simulink model "sim_ROV_v0_R2018b"  (R2023a)
settings: Solver=ode4  StartTime=0.0  StopTime=sim_time  FixedStep=Ts  RelTol=1e-3
values from neighbouring files (symbols this model uses):
  B = rho*V*g*1.4    (= 168.9282)    [launcher_ROV_sim.m]    (also in lqr_design.m = [0.05581,         0,         0,         0,         0,       )
  D_linear = diag([D_u, D_v, D_w, D_p, D_q, D_r])    [launcher_ROV_sim.m]
  D_quadratic = diag([D_uu, D_vv, D_ww, D_pp, D_qq, D_rr])    [launcher_ROV_sim.m]
  force = lookup.Force_14V_Kgf    [launcher_ROV_sim.m]
  I = [I_xx   -I_xy   -I_xz ... (first row only)    [launcher_ROV_sim.m]
  Kq = [-14.0522937866 -0.000724361189881 7.36173354264e-14 -0.00802187271501 -1.59153029576 -0.00240388685004 -0.00102573418256 -14.0209983601 3.7395785387e-14 1.84702452338 0.00611607698573 0.00818162190067 ... (36 elements, 6x6)]    [lqr.mat]    (also in lqr_design.m = K(:,13:end))
  Kx = [30.0077125539 0.00159520383282 -9.18372190817e-14 0.0101724452135 3.59932945814 0.00293162043647 0.00170650423442 25.0803818094 -2.91671924306e-14 -3.06896094423 -0.00658141948351 -0.00836683203268 ... (72 elements, 6x12)]    [lqr.mat]    (also in lqr_design.m = K(:,1:12))
  m = 16.6    [launcher_ROV_sim.m]
  M_addedMass = [1.3169    0         0         0         0         0 ... (first row only)    [launcher_ROV_sim.m]
  M_rigidBody = [m        0        0        0          m*z_g     -m*y_g ... (first row only)    [launcher_ROV_sim.m]
  pwm = lookup.PWM    [launcher_ROV_sim.m]
  r_b = [x_b y_b z_b]'    [launcher_ROV_sim.m]
  r_g = [x_g y_g z_g]'    [launcher_ROV_sim.m]
  sim_time = 100    [launcher_ROV_sim.m]    (also in lqr_design.m)
  TCM = [ -0.7071   -0.7071    0.7071    0.7071    0         0         0         0 ... (first row only)    [launcher_ROV_sim.m]
  Ts = 0.01    [launcher_ROV_sim.m]    (also in lqr_design.m)
  W = m*g    (= 162.846)    [launcher_ROV_sim.m]
libraries: slpidlib x6, dspfdesign x6, simulink x2, aerolibnav x1, sharedtransform x1, aerolibanim x1
(part 1 of 2)
settings Model: SimulationMode=accelerator  Creator=d066103  LastModifiedBy=retr0
settings SolverCC: AlgebraicLoopSolver=TrustRegion
settings DataIOCC: ReturnWorkspaceOutputs=off
settings DebuggingCC: UnconnectedInputMsg=warning  UnconnectedOutputMsg=warning  UnconnectedLineMsg=warning  ArithmeticOperatorsInVariantConditions=warning
settings HardwareCC: ProdBitPerPointer=32  ProdBitPerSizeT=32  ProdBitPerPtrDiffT=32  ProdLargestAtomicInteger=Long  ProdLargestAtomicFloat=Double  ProdWordSize=32  ProdHWDeviceType=ARM Compatible->ARM Cortex-M
settings ModelReferenceCC: EnableRefExpFcnMdlSchedulingChecks=on
settings SFSimCC: CustomCodeUndefinedFunction=UseInterfaceOnly
settings RTWCC: PackageGeneratedCodeAndArtifacts=on  TargetLang=C++
settings GRTTargetCC: TargetLangStandard=C++11 (ISO)

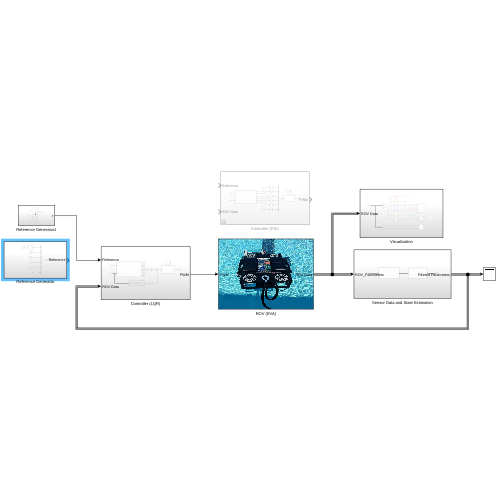
[thumbnail: Simulink's stored preview of the top-level diagram]
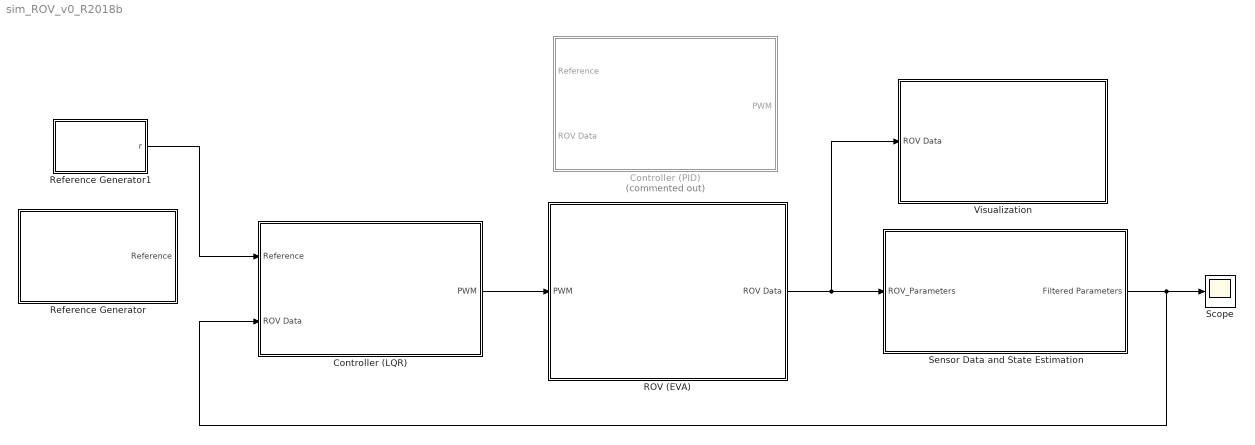
== system sim_ROV_v0_R2018b ==
  Controller (LQR) : Subsystem
  Controller (PID) : Subsystem  Commented=on
  ROV (EVA) : Subsystem
      mask Display: image('eva.jpg');
  Reference Generator : Subsystem
  Reference Generator1 : Subsystem
  Scope : Scope
  Sensor Data and State Estimation : Subsystem
  Visualization : Subsystem
  wires:
  ROV (EVA)/1(ROV Data) -> Visualization/1(ROV Data), Sensor Data and State Estimation/1(ROV_Parameters)
  Reference Generator1/1(r) -> Controller (LQR)/1(Reference)
  Controller (LQR)/1(PWM) -> ROV (EVA)/1(PWM)
  Sensor Data and State Estimation/1(Filtered Parameters) -> Scope/1, Controller (LQR)/2(ROV Data)

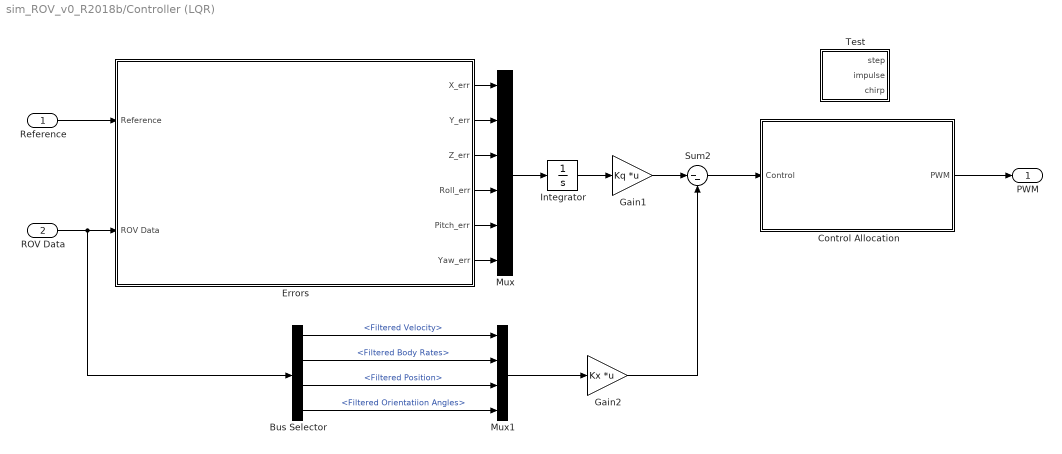
== system sim_ROV_v0_R2018b/Controller (LQR) ==
  Reference : Inport
  ROV Data : Inport  Port=2
  Bus Selector : BusSelector  OutputSignals=Filtered Velocity,Filtered Body Rates,Filtered Position,Filtered Orientatiion Angles
  Control Allocation : Subsystem
  Errors : Subsystem
  Gain1 : Gain  Gain=Kq  Multiplication=Matrix(K*u)
  Gain2 : Gain  Gain=Kx  Multiplication=Matrix(K*u)
  Integrator : Integrator
  Mux : Mux  Inputs=6
  Mux1 : Mux
  Sum2 : Sum  Inputs=|--
  Test : Subsystem
  PWM : Outport  VectorParamsAs1DForOutWhenUnconnected=off
  wires:
  Control Allocation/1(PWM) -> PWM/1
  Reference/1 -> Errors/1(Reference)
  ROV Data/1 -> Bus Selector/1, Errors/2(ROV Data)
  Errors/6(Yaw_err) -> Mux/6
  Errors/5(Pitch_err) -> Mux/5
  Errors/4(Roll_err) -> Mux/4
  Errors/3(Z_err) -> Mux/3
  Errors/2(Y_err) -> Mux/2
  Errors/1(X_err) -> Mux/1
  Mux/1 -> Integrator/1
  Gain1/1 -> Sum2/1
  Sum2/1 -> Control Allocation/1(Control)
  Gain2/1 -> Sum2/2
  Mux1/1 -> Gain2/1
  Bus Selector/2 -> Mux1/2  "<Filtered Body Rates>"
  Integrator/1 -> Gain1/1
  Bus Selector/3 -> Mux1/3  "<Filtered Position>"
  Bus Selector/4 -> Mux1/4  "<Filtered Orientatiion Angles>"
  Bus Selector/1 -> Mux1/1  "<Filtered Velocity>"

== system sim_ROV_v0_R2018b/Controller (PID) ==
  Reference : Inport
  ROV Data : Inport  Port=2
  Control Allocation : Subsystem
  Controller Pitch : slpidlib/PID Controller  Controller=PID  Form=Ideal  TimeDomain=Continuous-time  UseExternalTs=off  SampleTime=-1  IntegratorMethod=Forward Euler  FilterMethod=Forward Euler  ControllerParametersSource=internal  P=137.468345289691  I=0.00452061904362843  UseKiTs=off  D=0.10598803802833  N=59.0701245414644  UseFilter=on  TunerSelectOption=Transfer Function Based (PID Tuner App)  InitialConditionSource=internal  InitialConditionForIntegrator=0  InitialConditionForFilter=0  DifferentiatorICPrevScaledInput=0  ExternalReset=none  TrackingMode=off  Kt=1  LimitOutput=off  SatLimitsSource=internal  UpperSaturationLimit=inf  LowerSaturationLimit=-inf  LinearizeAsGain=on  AntiWindupMode=none  Kb=1  LimitIntegrator=off  UpperIntegratorSaturationLimit=inf  LowerIntegratorSaturationLimit=-inf  POutMin=[]  POutMax=[]  IOutMin=[]  IOutMax=[]  DOutMin=[]  DOutMax=[]  NOutMin=[]  NOutMax=[]  SumOutMin=[]  SumOutMax=[]  SaturationOutMin=[]  SaturationOutMax=[]  PParamMin=[]  PParamMax=[]  IParamMin=[]  IParamMax=[]  DParamMin=[]  DParamMax=[]  NParamMin=[]  NParamMax=[]  KbParamMin=[]  KbParamMax=[]  KtParamMin=[]  KtParamMax=[]  KbOutMin=[]  KbOutMax=[]  KtOutMin=[]  KtOutMax=[]  IntegratorOutMin=[]  IntegratorOutMax=[]  FilterOutMin=[]  FilterOutMax=[]  SumI1OutMin=[]  SumI1OutMax=[]  SumI2OutMin=[]  SumI2OutMax=[]  SumI3OutMin=[]  SumI3OutMax=[]  SumI4OutMin=[]  SumI4OutMax=[]  SumDOutMin=[]  SumDOutMax=[]  DifferentiatorOutMin=[]  DifferentiatorOutMax=[]  FilterDiffOutCoefMin=[]  FilterDiffOutCoefMax=[]  ReciprocalOutMin=[]  ReciprocalOutMax=[]  SumDenOutMin=[]  SumDenOutMax=[]  SumNumOutMin=[]  SumNumOutMax=[]  DivideOutMin=[]  DivideOutMax=[]  UdiffTsProdOutMin=[]  UdiffTsProdOutMax=[]  NTsProdOutMin=[]  NTsProdOutMax=[]  UintegralTsProdOutMin=[]  UintegralTsProdOutMax=[]  UngainTsProdOutMin=[]  UngainTsProdOutMax=[]  ClampingZeroOutDataTypeStr=Inherit: Inherit via back propagation  ClampingZeroOutMin=[]  ClampingZeroOutMax=[]  FilterDenConstantOutDataTypeStr=Inherit: Inherit via back propagation  FilterDenConstantOutMin=[]  FilterDenConstantOutMax=[]  PCopyOutDataTypeStr=Inherit: Inherit via back propagation  PCopyOutMin=[]  PCopyOutMax=[]  NCopyOutDataTypeStr=Inherit: Inherit via back propagation  NCopyOutMin=[]  NCopyOutMax=[]  IntegratorContinuousStateAttributes=''  IntegratorStateMustResolveToSignalObject=off  IntegratorRTWStateStorageClass=Auto  FilterContinuousStateAttributes=''  FilterStateMustResolveToSignalObject=off  FilterRTWStateStorageClass=Auto  ParallelPVariant=Passthrough  IdealPVariant=InternalParameters  IVariant=InternalParameters  DVariant=InternalParameters  IntegratorVariant=Continuous  SatVariant=Disabled  AWVariant=Passthrough  PCopyVariant=Disabled  TRVariant=Disabled  FdbkBlocksVariant=Forward  IdealPFdbkVariant=Disabled  SatFdbkVariant=Disabled  DerivativeFilterVariant=ContFilter  NVariant=InternalParameters  NCopyVariant=Disabled  FilterICVariant=InternalICsFilter  IntegratorICVariant=InternalICs  ExternalResetVariant=Disabled  TRSumVariant=Passthrough  SumFdbkVariant=Disabled  SumVariant=Sum_PID  TsampFilterVariant=InternalTs  TsampNgainVariant=Passthrough  TsampIntegralVariant=Disabled_SignalSpec  ExternalSaturationOutDataTypeStr=Inherit: Same as second input
  Controller Roll : slpidlib/PID Controller  Controller=PD  Form=Ideal  TimeDomain=Continuous-time  UseExternalTs=off  SampleTime=-1  IntegratorMethod=Forward Euler  FilterMethod=Forward Euler  ControllerParametersSource=internal  P=338.734488453615  I=0.00899012295658062  UseKiTs=off  D=0.0949817527302428  N=190.888436374434  UseFilter=on  TunerSelectOption=Transfer Function Based (PID Tuner App)  InitialConditionSource=internal  InitialConditionForIntegrator=0  InitialConditionForFilter=0  DifferentiatorICPrevScaledInput=0  ExternalReset=none  TrackingMode=off  Kt=1  LimitOutput=off  SatLimitsSource=internal  UpperSaturationLimit=inf  LowerSaturationLimit=-inf  LinearizeAsGain=on  AntiWindupMode=none  Kb=1  LimitIntegrator=off  UpperIntegratorSaturationLimit=inf  LowerIntegratorSaturationLimit=-inf  POutMin=[]  POutMax=[]  IOutMin=[]  IOutMax=[]  DOutMin=[]  DOutMax=[]  NOutMin=[]  NOutMax=[]  SumOutMin=[]  SumOutMax=[]  SaturationOutMin=[]  SaturationOutMax=[]  PParamMin=[]  PParamMax=[]  IParamMin=[]  IParamMax=[]  DParamMin=[]  DParamMax=[]  NParamMin=[]  NParamMax=[]  KbParamMin=[]  KbParamMax=[]  KtParamMin=[]  KtParamMax=[]  KbOutMin=[]  KbOutMax=[]  KtOutMin=[]  KtOutMax=[]  IntegratorOutMin=[]  IntegratorOutMax=[]  FilterOutMin=[]  FilterOutMax=[]  SumI1OutMin=[]  SumI1OutMax=[]  SumI2OutMin=[]  SumI2OutMax=[]  SumI3OutMin=[]  SumI3OutMax=[]  SumI4OutMin=[]  SumI4OutMax=[]  SumDOutMin=[]  SumDOutMax=[]  DifferentiatorOutMin=[]  DifferentiatorOutMax=[]  FilterDiffOutCoefMin=[]  FilterDiffOutCoefMax=[]  ReciprocalOutMin=[]  ReciprocalOutMax=[]  SumDenOutMin=[]  SumDenOutMax=[]  SumNumOutMin=[]  SumNumOutMax=[]  DivideOutMin=[]  DivideOutMax=[]  UdiffTsProdOutMin=[]  UdiffTsProdOutMax=[]  NTsProdOutMin=[]  NTsProdOutMax=[]  UintegralTsProdOutMin=[]  UintegralTsProdOutMax=[]  UngainTsProdOutMin=[]  UngainTsProdOutMax=[]  ClampingZeroOutDataTypeStr=Inherit: Inherit via back propagation  ClampingZeroOutMin=[]  ClampingZeroOutMax=[]  FilterDenConstantOutDataTypeStr=Inherit: Inherit via back propagation  FilterDenConstantOutMin=[]  FilterDenConstantOutMax=[]  PCopyOutDataTypeStr=Inherit: Inherit via back propagation  PCopyOutMin=[]  PCopyOutMax=[]  NCopyOutDataTypeStr=Inherit: Inherit via back propagation  NCopyOutMin=[]  NCopyOutMax=[]  IntegratorContinuousStateAttributes=''  IntegratorStateMustResolveToSignalObject=off  IntegratorRTWStateStorageClass=Auto  FilterContinuousStateAttributes=''  FilterStateMustResolveToSignalObject=off  FilterRTWStateStorageClass=Auto  ParallelPVariant=Passthrough  IdealPVariant=InternalParameters  IVariant=Disabled  DVariant=InternalParameters  IntegratorVariant=Disabled  SatVariant=Disabled  AWVariant=Disabled  PCopyVariant=Disabled  TRVariant=Disabled  FdbkBlocksVariant=Forward  IdealPFdbkVariant=Disabled  SatFdbkVariant=Disabled  DerivativeFilterVariant=ContFilter  NVariant=InternalParameters  NCopyVariant=Disabled  FilterICVariant=InternalICsFilter  IntegratorICVariant=Disabled  ExternalResetVariant=Disabled  TRSumVariant=Passthrough  SumFdbkVariant=Disabled  SumVariant=Sum_PD  TsampFilterVariant=InternalTs  TsampNgainVariant=Passthrough  TsampIntegralVariant=Disabled_SignalSpec  ExternalSaturationOutDataTypeStr=Inherit: Same as second input
  Controller X : slpidlib/PID Controller  Controller=PD  Form=Ideal  TimeDomain=Continuous-time  UseExternalTs=off  SampleTime=-1  IntegratorMethod=Forward Euler  FilterMethod=Forward Euler  ControllerParametersSource=internal  P=26.505422427304  I=0.00899012295658062  UseKiTs=off  D=0.620337341254882  N=0.955497663107341  UseFilter=on  TunerSelectOption=Transfer Function Based (PID Tuner App)  InitialConditionSource=internal  InitialConditionForIntegrator=0  InitialConditionForFilter=0  DifferentiatorICPrevScaledInput=0  ExternalReset=none  TrackingMode=off  Kt=1  LimitOutput=off  SatLimitsSource=internal  UpperSaturationLimit=inf  LowerSaturationLimit=-inf  LinearizeAsGain=on  AntiWindupMode=none  Kb=1  LimitIntegrator=off  UpperIntegratorSaturationLimit=inf  LowerIntegratorSaturationLimit=-inf  POutMin=[]  POutMax=[]  IOutMin=[]  IOutMax=[]  DOutMin=[]  DOutMax=[]  NOutMin=[]  NOutMax=[]  SumOutMin=[]  SumOutMax=[]  SaturationOutMin=[]  SaturationOutMax=[]  PParamMin=[]  PParamMax=[]  IParamMin=[]  IParamMax=[]  DParamMin=[]  DParamMax=[]  NParamMin=[]  NParamMax=[]  KbParamMin=[]  KbParamMax=[]  KtParamMin=[]  KtParamMax=[]  KbOutMin=[]  KbOutMax=[]  KtOutMin=[]  KtOutMax=[]  IntegratorOutMin=[]  IntegratorOutMax=[]  FilterOutMin=[]  FilterOutMax=[]  SumI1OutMin=[]  SumI1OutMax=[]  SumI2OutMin=[]  SumI2OutMax=[]  SumI3OutMin=[]  SumI3OutMax=[]  SumI4OutMin=[]  SumI4OutMax=[]  SumDOutMin=[]  SumDOutMax=[]  DifferentiatorOutMin=[]  DifferentiatorOutMax=[]  FilterDiffOutCoefMin=[]  FilterDiffOutCoefMax=[]  ReciprocalOutMin=[]  ReciprocalOutMax=[]  SumDenOutMin=[]  SumDenOutMax=[]  SumNumOutMin=[]  SumNumOutMax=[]  DivideOutMin=[]  DivideOutMax=[]  UdiffTsProdOutMin=[]  UdiffTsProdOutMax=[]  NTsProdOutMin=[]  NTsProdOutMax=[]  UintegralTsProdOutMin=[]  UintegralTsProdOutMax=[]  UngainTsProdOutMin=[]  UngainTsProdOutMax=[]  ClampingZeroOutDataTypeStr=Inherit: Inherit via back propagation  ClampingZeroOutMin=[]  ClampingZeroOutMax=[]  FilterDenConstantOutDataTypeStr=Inherit: Inherit via back propagation  FilterDenConstantOutMin=[]  FilterDenConstantOutMax=[]  PCopyOutDataTypeStr=Inherit: Inherit via back propagation  PCopyOutMin=[]  PCopyOutMax=[]  NCopyOutDataTypeStr=Inherit: Inherit via back propagation  NCopyOutMin=[]  NCopyOutMax=[]  IntegratorContinuousStateAttributes=''  IntegratorStateMustResolveToSignalObject=off  IntegratorRTWStateStorageClass=Auto  FilterContinuousStateAttributes=''  FilterStateMustResolveToSignalObject=off  FilterRTWStateStorageClass=Auto  ParallelPVariant=Passthrough  IdealPVariant=InternalParameters  IVariant=Disabled  DVariant=InternalParameters  IntegratorVariant=Disabled  SatVariant=Disabled  AWVariant=Disabled  PCopyVariant=Disabled  TRVariant=Disabled  FdbkBlocksVariant=Forward  IdealPFdbkVariant=Disabled  SatFdbkVariant=Disabled  DerivativeFilterVariant=ContFilter  NVariant=InternalParameters  NCopyVariant=Disabled  FilterICVariant=InternalICsFilter  IntegratorICVariant=Disabled  ExternalResetVariant=Disabled  TRSumVariant=Passthrough  SumFdbkVariant=Disabled  SumVariant=Sum_PD  TsampFilterVariant=InternalTs  TsampNgainVariant=Passthrough  TsampIntegralVariant=Disabled_SignalSpec  ExternalSaturationOutDataTypeStr=Inherit: Same as second input
  Controller Y : slpidlib/PID Controller  Controller=PD  Form=Ideal  TimeDomain=Continuous-time  UseExternalTs=off  SampleTime=-1  IntegratorMethod=Forward Euler  FilterMethod=Forward Euler  ControllerParametersSource=internal  P=54.0411515772124  I=0.00335999548481141  UseKiTs=off  D=3.50685578049318  N=0.462269774575205  UseFilter=on  TunerSelectOption=Transfer Function Based (PID Tuner App)  InitialConditionSource=internal  InitialConditionForIntegrator=0  InitialConditionForFilter=0  DifferentiatorICPrevScaledInput=0  ExternalReset=none  TrackingMode=off  Kt=1  LimitOutput=off  SatLimitsSource=internal  UpperSaturationLimit=inf  LowerSaturationLimit=-inf  LinearizeAsGain=on  AntiWindupMode=none  Kb=1  LimitIntegrator=off  UpperIntegratorSaturationLimit=inf  LowerIntegratorSaturationLimit=-inf  POutMin=[]  POutMax=[]  IOutMin=[]  IOutMax=[]  DOutMin=[]  DOutMax=[]  NOutMin=[]  NOutMax=[]  SumOutMin=[]  SumOutMax=[]  SaturationOutMin=[]  SaturationOutMax=[]  PParamMin=[]  PParamMax=[]  IParamMin=[]  IParamMax=[]  DParamMin=[]  DParamMax=[]  NParamMin=[]  NParamMax=[]  KbParamMin=[]  KbParamMax=[]  KtParamMin=[]  KtParamMax=[]  KbOutMin=[]  KbOutMax=[]  KtOutMin=[]  KtOutMax=[]  IntegratorOutMin=[]  IntegratorOutMax=[]  FilterOutMin=[]  FilterOutMax=[]  SumI1OutMin=[]  SumI1OutMax=[]  SumI2OutMin=[]  SumI2OutMax=[]  SumI3OutMin=[]  SumI3OutMax=[]  SumI4OutMin=[]  SumI4OutMax=[]  SumDOutMin=[]  SumDOutMax=[]  DifferentiatorOutMin=[]  DifferentiatorOutMax=[]  FilterDiffOutCoefMin=[]  FilterDiffOutCoefMax=[]  ReciprocalOutMin=[]  ReciprocalOutMax=[]  SumDenOutMin=[]  SumDenOutMax=[]  SumNumOutMin=[]  SumNumOutMax=[]  DivideOutMin=[]  DivideOutMax=[]  UdiffTsProdOutMin=[]  UdiffTsProdOutMax=[]  NTsProdOutMin=[]  NTsProdOutMax=[]  UintegralTsProdOutMin=[]  UintegralTsProdOutMax=[]  UngainTsProdOutMin=[]  UngainTsProdOutMax=[]  ClampingZeroOutDataTypeStr=Inherit: Inherit via back propagation  ClampingZeroOutMin=[]  ClampingZeroOutMax=[]  FilterDenConstantOutDataTypeStr=Inherit: Inherit via back propagation  FilterDenConstantOutMin=[]  FilterDenConstantOutMax=[]  PCopyOutDataTypeStr=Inherit: Inherit via back propagation  PCopyOutMin=[]  PCopyOutMax=[]  NCopyOutDataTypeStr=Inherit: Inherit via back propagation  NCopyOutMin=[]  NCopyOutMax=[]  IntegratorContinuousStateAttributes=''  IntegratorStateMustResolveToSignalObject=off  IntegratorRTWStateStorageClass=Auto  FilterContinuousStateAttributes=''  FilterStateMustResolveToSignalObject=off  FilterRTWStateStorageClass=Auto  ParallelPVariant=Passthrough  IdealPVariant=InternalParameters  IVariant=Disabled  DVariant=InternalParameters  IntegratorVariant=Disabled  SatVariant=Disabled  AWVariant=Disabled  PCopyVariant=Disabled  TRVariant=Disabled  FdbkBlocksVariant=Forward  IdealPFdbkVariant=Disabled  SatFdbkVariant=Disabled  DerivativeFilterVariant=ContFilter  NVariant=InternalParameters  NCopyVariant=Disabled  FilterICVariant=InternalICsFilter  IntegratorICVariant=Disabled  ExternalResetVariant=Disabled  TRSumVariant=Passthrough  SumFdbkVariant=Disabled  SumVariant=Sum_PD  TsampFilterVariant=InternalTs  TsampNgainVariant=Passthrough  TsampIntegralVariant=Disabled_SignalSpec  ExternalSaturationOutDataTypeStr=Inherit: Same as second input
  Controller Yaw : slpidlib/PID Controller  Controller=PID  Form=Ideal  TimeDomain=Continuous-time  UseExternalTs=off  SampleTime=-1  IntegratorMethod=Forward Euler  FilterMethod=Forward Euler  ControllerParametersSource=internal  P=0.0221243978398075  I=0.00101259882844407  UseKiTs=off  D=107.142129388811  N=15.0943187295303  UseFilter=on  TunerSelectOption=Transfer Function Based (PID Tuner App)  InitialConditionSource=internal  InitialConditionForIntegrator=0  InitialConditionForFilter=0  DifferentiatorICPrevScaledInput=0  ExternalReset=none  TrackingMode=off  Kt=1  LimitOutput=off  SatLimitsSource=internal  UpperSaturationLimit=inf  LowerSaturationLimit=-inf  LinearizeAsGain=on  AntiWindupMode=none  Kb=1  LimitIntegrator=off  UpperIntegratorSaturationLimit=inf  LowerIntegratorSaturationLimit=-inf  POutMin=[]  POutMax=[]  IOutMin=[]  IOutMax=[]  DOutMin=[]  DOutMax=[]  NOutMin=[]  NOutMax=[]  SumOutMin=[]  SumOutMax=[]  SaturationOutMin=[]  SaturationOutMax=[]  PParamMin=[]  PParamMax=[]  IParamMin=[]  IParamMax=[]  DParamMin=[]  DParamMax=[]  NParamMin=[]  NParamMax=[]  KbParamMin=[]  KbParamMax=[]  KtParamMin=[]  KtParamMax=[]  KbOutMin=[]  KbOutMax=[]  KtOutMin=[]  KtOutMax=[]  IntegratorOutMin=[]  IntegratorOutMax=[]  FilterOutMin=[]  FilterOutMax=[]  SumI1OutMin=[]  SumI1OutMax=[]  SumI2OutMin=[]  SumI2OutMax=[]  SumI3OutMin=[]  SumI3OutMax=[]  SumI4OutMin=[]  SumI4OutMax=[]  SumDOutMin=[]  SumDOutMax=[]  DifferentiatorOutMin=[]  DifferentiatorOutMax=[]  FilterDiffOutCoefMin=[]  FilterDiffOutCoefMax=[]  ReciprocalOutMin=[]  ReciprocalOutMax=[]  SumDenOutMin=[]  SumDenOutMax=[]  SumNumOutMin=[]  SumNumOutMax=[]  DivideOutMin=[]  DivideOutMax=[]  UdiffTsProdOutMin=[]  UdiffTsProdOutMax=[]  NTsProdOutMin=[]  NTsProdOutMax=[]  UintegralTsProdOutMin=[]  UintegralTsProdOutMax=[]  UngainTsProdOutMin=[]  UngainTsProdOutMax=[]  ClampingZeroOutDataTypeStr=Inherit: Inherit via back propagation  ClampingZeroOutMin=[]  ClampingZeroOutMax=[]  FilterDenConstantOutDataTypeStr=Inherit: Inherit via back propagation  FilterDenConstantOutMin=[]  FilterDenConstantOutMax=[]  PCopyOutDataTypeStr=Inherit: Inherit via back propagation  PCopyOutMin=[]  PCopyOutMax=[]  NCopyOutDataTypeStr=Inherit: Inherit via back propagation  NCopyOutMin=[]  NCopyOutMax=[]  IntegratorContinuousStateAttributes=''  IntegratorStateMustResolveToSignalObject=off  IntegratorRTWStateStorageClass=Auto  FilterContinuousStateAttributes=''  FilterStateMustResolveToSignalObject=off  FilterRTWStateStorageClass=Auto  ParallelPVariant=Passthrough  IdealPVariant=InternalParameters  IVariant=InternalParameters  DVariant=InternalParameters  IntegratorVariant=Continuous  SatVariant=Disabled  AWVariant=Passthrough  PCopyVariant=Disabled  TRVariant=Disabled  FdbkBlocksVariant=Forward  IdealPFdbkVariant=Disabled  SatFdbkVariant=Disabled  DerivativeFilterVariant=ContFilter  NVariant=InternalParameters  NCopyVariant=Disabled  FilterICVariant=InternalICsFilter  IntegratorICVariant=InternalICs  ExternalResetVariant=Disabled  TRSumVariant=Passthrough  SumFdbkVariant=Disabled  SumVariant=Sum_PID  TsampFilterVariant=InternalTs  TsampNgainVariant=Passthrough  TsampIntegralVariant=Disabled_SignalSpec  ExternalSaturationOutDataTypeStr=Inherit: Same as second input
  Controller Z : slpidlib/PID Controller  Controller=PID  Form=Ideal  TimeDomain=Discrete-time  UseExternalTs=off  SampleTime=-1  IntegratorMethod=Forward Euler  FilterMethod=Forward Euler  ControllerParametersSource=internal  P=150  I=20  UseKiTs=off  D=200  N=85  UseFilter=on  TunerSelectOption=Transfer Function Based (PID Tuner App)  InitialConditionSource=internal  InitialConditionForIntegrator=0  InitialConditionForFilter=0  DifferentiatorICPrevScaledInput=0  ExternalReset=none  TrackingMode=off  Kt=1  LimitOutput=off  SatLimitsSource=internal  UpperSaturationLimit=inf  LowerSaturationLimit=-inf  LinearizeAsGain=on  AntiWindupMode=none  Kb=1  LimitIntegrator=off  UpperIntegratorSaturationLimit=inf  LowerIntegratorSaturationLimit=-inf  POutMin=[]  POutMax=[]  IOutMin=[]  IOutMax=[]  DOutMin=[]  DOutMax=[]  NOutMin=[]  NOutMax=[]  SumOutMin=[]  SumOutMax=[]  SaturationOutMin=[]  SaturationOutMax=[]  PParamMin=[]  PParamMax=[]  IParamMin=[]  IParamMax=[]  DParamMin=[]  DParamMax=[]  NParamMin=[]  NParamMax=[]  KbParamMin=[]  KbParamMax=[]  KtParamMin=[]  KtParamMax=[]  KbOutMin=[]  KbOutMax=[]  KtOutMin=[]  KtOutMax=[]  IntegratorOutMin=[]  IntegratorOutMax=[]  FilterOutMin=[]  FilterOutMax=[]  SumI1OutMin=[]  SumI1OutMax=[]  SumI2OutMin=[]  SumI2OutMax=[]  SumI3OutMin=[]  SumI3OutMax=[]  SumI4OutMin=[]  SumI4OutMax=[]  SumDOutMin=[]  SumDOutMax=[]  DifferentiatorOutMin=[]  DifferentiatorOutMax=[]  FilterDiffOutCoefMin=[]  FilterDiffOutCoefMax=[]  ReciprocalOutMin=[]  ReciprocalOutMax=[]  SumDenOutMin=[]  SumDenOutMax=[]  SumNumOutMin=[]  SumNumOutMax=[]  DivideOutMin=[]  DivideOutMax=[]  UdiffTsProdOutMin=[]  UdiffTsProdOutMax=[]  NTsProdOutMin=[]  NTsProdOutMax=[]  UintegralTsProdOutMin=[]  UintegralTsProdOutMax=[]  UngainTsProdOutMin=[]  UngainTsProdOutMax=[]  ClampingZeroOutDataTypeStr=Inherit: Inherit via back propagation  ClampingZeroOutMin=[]  ClampingZeroOutMax=[]  FilterDenConstantOutDataTypeStr=Inherit: Inherit via back propagation  FilterDenConstantOutMin=[]  FilterDenConstantOutMax=[]  PCopyOutDataTypeStr=Inherit: Inherit via back propagation  PCopyOutMin=[]  PCopyOutMax=[]  NCopyOutDataTypeStr=Inherit: Inherit via back propagation  NCopyOutMin=[]  NCopyOutMax=[]  IntegratorContinuousStateAttributes=''  IntegratorStateMustResolveToSignalObject=off  IntegratorRTWStateStorageClass=Auto  FilterContinuousStateAttributes=''  FilterStateMustResolveToSignalObject=off  FilterRTWStateStorageClass=Auto  ParallelPVariant=Passthrough  IdealPVariant=InternalParameters  IVariant=InternalParameters  DVariant=InternalParameters  IntegratorVariant=Discrete  SatVariant=Disabled  AWVariant=Passthrough  PCopyVariant=Disabled  TRVariant=Disabled  FdbkBlocksVariant=Forward  IdealPFdbkVariant=Disabled  SatFdbkVariant=Disabled  DerivativeFilterVariant=ForwardEulerFilter  NVariant=InternalParameters  NCopyVariant=Disabled  FilterICVariant=InternalICsFilter  IntegratorICVariant=InternalICs  ExternalResetVariant=Disabled  TRSumVariant=Passthrough  SumFdbkVariant=Disabled  SumVariant=Sum_PID  TsampFilterVariant=InternalTs  TsampNgainVariant=Passthrough  TsampIntegralVariant=Disabled_SignalSpec  ExternalSaturationOutDataTypeStr=Inherit: Same as second input
  Errors : Subsystem
  Mux : Mux  Inputs=6
  Test : Subsystem
  PWM : Outport  VectorParamsAs1DForOutWhenUnconnected=off
  wires:
  Mux/1 -> Control Allocation/1(Control)
  Control Allocation/1(PWM) -> PWM/1
  Reference/1 -> Errors/1(Reference)
  ROV Data/1 -> Errors/2(ROV Data)
  Errors/1(X_err) -> Controller X/1
  Errors/3(Z_err) -> Controller Z/1
  Errors/4(Roll_err) -> Controller Roll/1
  Errors/6(Yaw_err) -> Controller Yaw/1
  Errors/5(Pitch_err) -> Controller Pitch/1
  Controller X/1 -> Mux/1
  Controller Z/1 -> Mux/3
  Controller Roll/1 -> Mux/4
  Controller Pitch/1 -> Mux/5
  Controller Yaw/1 -> Mux/6
  Controller Y/1 -> Mux/2
  Errors/2(Y_err) -> Controller Y/1

== system sim_ROV_v0_R2018b/ROV (EVA) ==
  PWM : Inport
  Actuators Dynamics : Subsystem
      mask Display: image('t200.jpg');
  Bus Creator : BusCreator  Inputs=2
  Post-Processing : Subsystem
  ROV (non-linear) : Subsystem  Commented=on
  Rigid Body Dynamics : Subsystem
  Rigid Body Kinematics : Subsystem
  Thrust Configuration Matrix : Gain  Gain=TCM  Multiplication=Matrix(K*u)
  ROV Data : Outport  VectorParamsAs1DForOutWhenUnconnected=off
  wires:
  PWM/1 -> Actuators Dynamics/1(PWM)
  Rigid Body Dynamics/1(Kinematics (Body)) -> Post-Processing/3(Kinematics (Body)), Rigid Body Kinematics/1(Kinematics (Body))
  Rigid Body Kinematics/1(Kinematics (Fixed)) -> Post-Processing/2(Kinematics (Fixed))
  Bus Creator/1 -> Post-Processing/1(Porpulsion)  "Propulsion"
  Thrust Configuration Matrix/1 -> Rigid Body Dynamics/1(Forces & Moments), Bus Creator/2  "Forces & Moments"
  Actuators Dynamics/1(Thrust (N)) -> Bus Creator/1, Thrust Configuration Matrix/1  "Actuators Thrusts"
  Post-Processing/1(ROV Data) -> Rigid Body Dynamics/2(ROV Data), ROV Data/1

== system sim_ROV_v0_R2018b/Reference Generator ==
  Gain : Gain  Gain=pi/180
  Gain1 : Gain  Gain=pi/180
  Gain2 : Gain  Gain=pi/180
  Mux : Mux  Inputs=6
  Reference Pitch : Constant  Value=0
  Reference Roll : Constant  Value=0
  Reference X : Constant  Value=40
  Reference Y : Constant  Value=0
  Reference Yaw : Constant  Value=0
  Reference Z : Constant
  Step : Subsystem
  Reference : Outport  VectorParamsAs1DForOutWhenUnconnected=off
  wires:
  Mux/1 -> Reference/1
  Reference Y/1 -> Mux/2
  Reference Z/1 -> Mux/3
  Reference Pitch/1 -> Gain1/1
  Reference Yaw/1 -> Gain2/1
  Reference Roll/1 -> Gain/1
  Gain/1 -> Mux/4
  Gain1/1 -> Mux/5
  Gain2/1 -> Mux/6
  Step/1(step) -> Mux/1

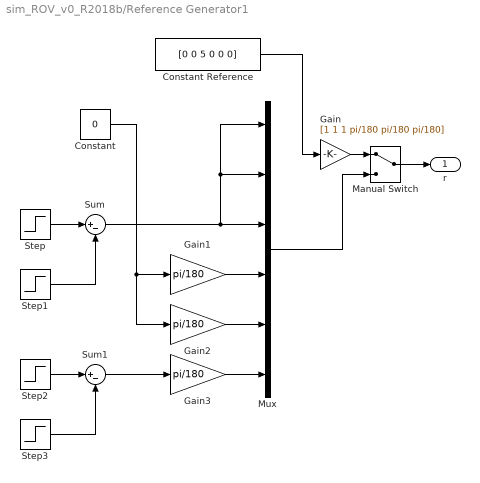
== system sim_ROV_v0_R2018b/Reference Generator1 ==
  Constant : Constant  Value=0
  Constant Reference : Constant  Value=[0 0 5 0 0 0]
  Gain : Gain  Gain=[1 1 1 pi/180 pi/180 pi/180]
  Gain1 : Gain  Gain=pi/180
  Gain2 : Gain  Gain=pi/180
  Gain3 : Gain  Gain=pi/180
  Manual Switch : ManualSwitch
  Mux : Mux  Inputs=6
  Step : Step  Time=10  After=5  SampleTime=0
  Step1 : Step  Time=60  After=5  SampleTime=0
  Step2 : Step  Time=10  After=90  SampleTime=0
  Step3 : Step  Time=60  After=90  SampleTime=0
  Sum : Sum  Inputs=|+-
  Sum1 : Sum  Inputs=|+-
  r : Outport  VectorParamsAs1DForOutWhenUnconnected=off
  wires:
  Constant Reference/1 -> Gain/1
  Manual Switch/1 -> r/1
  Mux/1 -> Manual Switch/2
  Sum/1 -> Mux/1, Mux/2, Mux/3
  Constant/1 -> Gain1/1, Gain2/1
  Step/1 -> Sum/1
  Step1/1 -> Sum/2
  Gain/1 -> Manual Switch/1
  Gain1/1 -> Mux/4
  Gain2/1 -> Mux/5
  Gain3/1 -> Mux/6
  Step3/1 -> Sum1/2
  Step2/1 -> Sum1/1
  Sum1/1 -> Gain3/1

== system sim_ROV_v0_R2018b/Sensor Data and State Estimation ==
  ROV_Parameters : Inport
  Internal Filter : Subsystem
  Sensor (IMU) : Subsystem
  Filtered Parameters : Outport  VectorParamsAs1DForOutWhenUnconnected=off
  wires:
  ROV_Parameters/1 -> Sensor (IMU)/1(IMU Inputs)
  Sensor (IMU)/1(IMU Measurements) -> Internal Filter/1(IMU Measurements)
  Internal Filter/1(Filtered Parameters) -> Filtered Parameters/1

== system sim_ROV_v0_R2018b/Visualization ==
  ROV Data : Inport
  3D Animation : Subsystem  Commented=on
  6DoF Animation : aerolibanim/6DoF Animation  u1=[-25 25 -25 25 -25 25]  u2=10*Ts  u3=20  u4=[5000 5000 5000]  u5=Fixed position  u6=[200 250 -200]  u7=10  u8=on
  Angular Acceleration : Selector  InputPortWidth=6  IndexOptions=Index vector (dialog)  Indices=[4:6]  OutputSizes=1
  Angular Velocity : Selector  InputPortWidth=6  IndexOptions=Index vector (dialog)  Indices=[4:6]  OutputSizes=1
  Attitude : Selector  InputPortWidth=6  IndexOptions=Index vector (dialog)  Indices=[4:6]  OutputSizes=1
  Bus Selector : BusSelector  OutputSignals=Kinematics (Fixed).Acceleration,Kinematics (Fixed).Velocity,Kinematics (Fixed).Pose
  Bus Selector1 : BusSelector  OutputSignals=Propulsion.Actuators Thrusts,Propulsion.Forces & Moments
  Linear Acceleration : Selector  InputPortWidth=6  IndexOptions=Index vector (dialog)  Indices=[1:3]  OutputSizes=1
  Linear Velocity : Selector  InputPortWidth=6  IndexOptions=Index vector (dialog)  Indices=[1:3]  OutputSizes=1
  Position : Selector  InputPortWidth=6  IndexOptions=Index vector (dialog)  Indices=[1:3]  OutputSizes=1
  Visualization (Kinematics) : Scope  NumInputPorts=6
  Visualization (Propulsion) : Scope  NumInputPorts=2
  wires:
  Bus Selector/3 -> Attitude/1, Position/1  "<Pose>"
  Bus Selector/2 -> Angular Velocity/1, Linear Velocity/1  "<Velocity>"
  Bus Selector/1 -> Angular Acceleration/1, Linear Acceleration/1  "<Acceleration>"
  Linear Acceleration/1 -> Visualization (Kinematics)/1
  Angular Acceleration/1 -> Visualization (Kinematics)/4
  Linear Velocity/1 -> Visualization (Kinematics)/2
  Angular Velocity/1 -> Visualization (Kinematics)/5
  ROV Data/1 -> Bus Selector1/1, Bus Selector/1
  Bus Selector1/1 -> Visualization (Propulsion)/1  "<Actuators Thrusts>"
  Bus Selector1/2 -> Visualization (Propulsion)/2  "<Forces & Moments>"
  Attitude/1 -> 6DoF Animation/2, Visualization (Kinematics)/6
  Position/1 -> 6DoF Animation/1, Visualization (Kinematics)/3

== system sim_ROV_v0_R2018b/Controller (LQR)/Control Allocation ==
  Control : Inport
  1-D Lookup Table : Lookup_n-D  NumberOfTableDimensions=1  BreakpointsForDimension1=force  Table=pwm  InternalRulePriority=Speed  RndMeth=Simplest
  Control Allocation : Gain  Gain=TCM'*inv(TCM*TCM')  Multiplication=Matrix(K*u)
  N → kgf : Gain  Gain=1/9.8
  Saturation : Saturate  UpperLimit=force(end)*9.8  LowerLimit=force(1)*9.8
  PWM : Outport  VectorParamsAs1DForOutWhenUnconnected=off
  wires:
  Control Allocation/1 -> Saturation/1  "Thrust (N)"
  Control/1 -> Control Allocation/1
  Saturation/1 -> N → kgf/1
  N → kgf/1 -> 1-D Lookup Table/1  "Thrust (kgf)"
  1-D Lookup Table/1 -> PWM/1

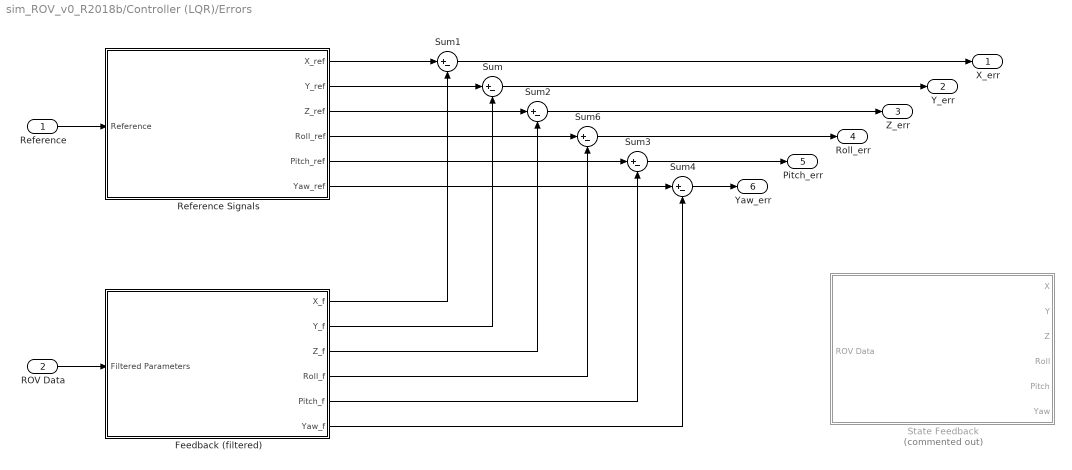
== system sim_ROV_v0_R2018b/Controller (LQR)/Errors ==
  Reference : Inport
  ROV Data : Inport  Port=2
  Feedback (filtered) : Subsystem
  Reference Signals : Subsystem
  State Feedback : Subsystem  Commented=on
  Sum{,1..4,6} (6 alike) : Sum  Inputs=|+-
  X_err : Outport  VectorParamsAs1DForOutWhenUnconnected=off
  Y_err : Outport  Port=2  VectorParamsAs1DForOutWhenUnconnected=off
  Z_err : Outport  Port=3  VectorParamsAs1DForOutWhenUnconnected=off
  Roll_err : Outport  Port=4  VectorParamsAs1DForOutWhenUnconnected=off
  Pitch_err : Outport  Port=5  VectorParamsAs1DForOutWhenUnconnected=off
  Yaw_err : Outport  Port=6  VectorParamsAs1DForOutWhenUnconnected=off
  wires:
  Sum1/1 -> X_err/1
  Sum2/1 -> Z_err/1
  Sum/1 -> Y_err/1
  Reference/1 -> Reference Signals/1(Reference)
  Reference Signals/1(X_ref) -> Sum1/1
  Reference Signals/2(Y_ref) -> Sum/1
  Reference Signals/3(Z_ref) -> Sum2/1
  Sum3/1 -> Pitch_err/1
  Reference Signals/5(Pitch_ref) -> Sum3/1
  Sum4/1 -> Yaw_err/1
  Reference Signals/6(Yaw_ref) -> Sum4/1
  Sum6/1 -> Roll_err/1
  Reference Signals/4(Roll_ref) -> Sum6/1
  ROV Data/1 -> Feedback (filtered)/1(Filtered Parameters)
  Feedback (filtered)/1(X_f) -> Sum1/2
  Feedback (filtered)/2(Y_f) -> Sum/2
  Feedback (filtered)/3(Z_f) -> Sum2/2
  Feedback (filtered)/4(Roll_f) -> Sum6/2
  Feedback (filtered)/5(Pitch_f) -> Sum3/2
  Feedback (filtered)/6(Yaw_f) -> Sum4/2

== system sim_ROV_v0_R2018b/Controller (LQR)/Test ==
  Chirp : Subsystem
  Impulse : Subsystem
  Step : Subsystem
  step : Outport  VectorParamsAs1DForOutWhenUnconnected=off
  impulse : Outport  Port=2  VectorParamsAs1DForOutWhenUnconnected=off
  chirp : Outport  Port=3  VectorParamsAs1DForOutWhenUnconnected=off
  wires:
  Step/1(step) -> step/1
  Impulse/1(impulse) -> impulse/1
  Chirp/1(chirp) -> chirp/1

== system sim_ROV_v0_R2018b/Controller (PID)/Control Allocation ==
  Control : Inport
  1-D Lookup Table : Lookup_n-D  NumberOfTableDimensions=1  BreakpointsForDimension1=force  Table=pwm  InternalRulePriority=Speed  RndMeth=Simplest
  Control Allocation : Gain  Gain=TCM'*inv(TCM*TCM')  Multiplication=Matrix(K*u)
  N → kgf : Gain  Gain=1/9.8
  Saturation : Saturate  UpperLimit=force(end)*9.8  LowerLimit=force(1)*9.8
  PWM : Outport  VectorParamsAs1DForOutWhenUnconnected=off
  wires:
  Control Allocation/1 -> Saturation/1  "Thrust (N)"
  Control/1 -> Control Allocation/1
  Saturation/1 -> N → kgf/1
  N → kgf/1 -> 1-D Lookup Table/1  "Thrust (kgf)"
  1-D Lookup Table/1 -> PWM/1

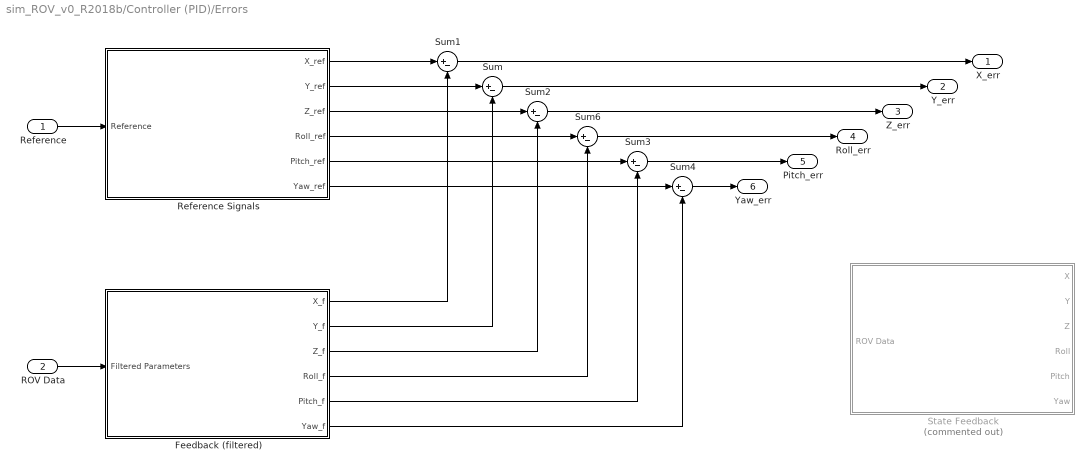
== system sim_ROV_v0_R2018b/Controller (PID)/Errors ==
  Reference : Inport
  ROV Data : Inport  Port=2
  Feedback (filtered) : Subsystem
  Reference Signals : Subsystem
  State Feedback : Subsystem  Commented=on
  Sum{,1..4,6} (6 alike) : Sum  Inputs=|+-
  X_err : Outport  VectorParamsAs1DForOutWhenUnconnected=off
  Y_err : Outport  Port=2  VectorParamsAs1DForOutWhenUnconnected=off
  Z_err : Outport  Port=3  VectorParamsAs1DForOutWhenUnconnected=off
  Roll_err : Outport  Port=4  VectorParamsAs1DForOutWhenUnconnected=off
  Pitch_err : Outport  Port=5  VectorParamsAs1DForOutWhenUnconnected=off
  Yaw_err : Outport  Port=6  VectorParamsAs1DForOutWhenUnconnected=off
  wires:
  Sum1/1 -> X_err/1
  Sum2/1 -> Z_err/1
  Sum/1 -> Y_err/1
  Reference/1 -> Reference Signals/1(Reference)
  Reference Signals/1(X_ref) -> Sum1/1
  Reference Signals/2(Y_ref) -> Sum/1
  Reference Signals/3(Z_ref) -> Sum2/1
  Sum3/1 -> Pitch_err/1
  Reference Signals/5(Pitch_ref) -> Sum3/1
  Sum4/1 -> Yaw_err/1
  Reference Signals/6(Yaw_ref) -> Sum4/1
  Sum6/1 -> Roll_err/1
  Reference Signals/4(Roll_ref) -> Sum6/1
  ROV Data/1 -> Feedback (filtered)/1(Filtered Parameters)
  Feedback (filtered)/1(X_f) -> Sum1/2
  Feedback (filtered)/2(Y_f) -> Sum/2
  Feedback (filtered)/3(Z_f) -> Sum2/2
  Feedback (filtered)/4(Roll_f) -> Sum6/2
  Feedback (filtered)/5(Pitch_f) -> Sum3/2
  Feedback (filtered)/6(Yaw_f) -> Sum4/2

== system sim_ROV_v0_R2018b/Controller (PID)/Test ==
  Chirp : Subsystem
  Impulse : Subsystem
  Step : Subsystem
  step : Outport  VectorParamsAs1DForOutWhenUnconnected=off
  impulse : Outport  Port=2  VectorParamsAs1DForOutWhenUnconnected=off
  chirp : Outport  Port=3  VectorParamsAs1DForOutWhenUnconnected=off
  wires:
  Step/1(step) -> step/1
  Impulse/1(impulse) -> impulse/1
  Chirp/1(chirp) -> chirp/1

== system sim_ROV_v0_R2018b/ROV (EVA)/Actuators Dynamics ==
  note: Blue Robotics T200 System Identification
  note: Since the input and output data used for the identification have been detrended and filtered we have to map the input
      | before providing it to the TF. Moreover the output used for the identification was in lbf, hence we have to convert it in N.
  PWM : Inport
  Dead Zone : DeadZone  LowerValue=-10  UpperValue=+10
  Motors Transfer Functions : Subsystem
  Normalization : MATLAB Function  TreatAsAtomicUnit=on
  Saturation : Saturate  UpperLimit=1900  LowerLimit=1100
  lbf → N : Gain  Gain=4.45
  Thrust (N) : Outport  VectorParamsAs1DForOutWhenUnconnected=off
  wires:
  Normalization/1(y) -> Dead Zone/1
  Saturation/1 -> Normalization/1(u)
  lbf → N/1 -> Thrust (N)/1  "Thrust (N)"
  PWM/1 -> Saturation/1
  Dead Zone/1 -> Motors Transfer Functions/1(pwm)
  Motors Transfer Functions/1(lbf) -> lbf → N/1

== system sim_ROV_v0_R2018b/ROV (EVA)/Post-Processing ==
  Porpulsion : Inport
  Kinematics (Fixed) : Inport  Port=2
  Kinematics (Body) : Inport  Port=3
  Body Angular Acceleration : Selector  InputPortWidth=6  IndexOptions=Index vector (dialog)  Indices=[4:6]  OutputSizes=1
  Body Angular Rates : Selector  InputPortWidth=6  IndexOptions=Index vector (dialog)  Indices=[4:6]  OutputSizes=1
  Body Linear Acceleration : Selector  InputPortWidth=6  IndexOptions=Index vector (dialog)  Indices=[1:3]  OutputSizes=1
  Bus Creator : BusCreator  Inputs=3
  Bus Selector : BusSelector  OutputSignals=Body Velocity,Body Acceleration
  CoG : Constant  Value=r_g
  Gravity Acceleration : Constant  Value=[0 0 0]
  Mux : Mux  Inputs=5
  ROV Data : Outport  VectorParamsAs1DForOutWhenUnconnected=off
  wires:
  Body Angular Rates/1 -> Mux/2
  CoG/1 -> Mux/4
  Body Angular Acceleration/1 -> Mux/3
  Mux/1 -> Bus Creator/3  "IMU Data"
  Gravity Acceleration/1 -> Mux/5
  Bus Creator/1 -> ROV Data/1
  Body Linear Acceleration/1 -> Mux/1
  Kinematics (Body)/1 -> Bus Selector/1
  Kinematics (Fixed)/1 -> Bus Creator/2  "Kinematics (Fixed)"
  Bus Selector/1 -> Body Angular Rates/1  "<Body Velocity>"
  Bus Selector/2 -> Body Linear Acceleration/1, Body Angular Acceleration/1  "<Body Acceleration>"
  Porpulsion/1 -> Bus Creator/1

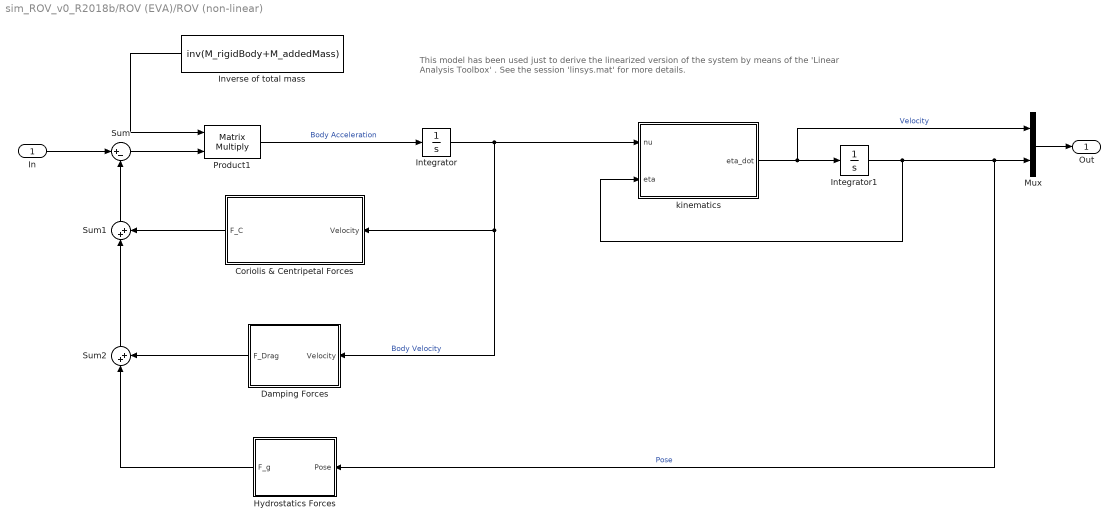
== system sim_ROV_v0_R2018b/ROV (EVA)/ROV (non-linear) ==
  note: This model has been used just to derive the linearized version of the system by means of the 'Linear Analysis Toolbox' .
      | See the session 'linsys.mat' for more details.
  In : Inport
  Coriolis & Centripetal Forces : Subsystem
  Damping Forces : Subsystem
  Hydrostatics Forces : Subsystem
  Integrator : Integrator
  Integrator1 : Integrator
  Inverse of total mass : Constant  Value=inv(M_rigidBody+M_addedMass)
  Mux : Mux  Inputs=2
  Product1 : Product  Multiplication=Matrix(*)  RndMeth=Zero
  Sum : Sum  Inputs=|+-
  Sum1 : Sum  Inputs=|++
  Sum2 : Sum  Inputs=|++
  kinematics : MATLAB Function  TreatAsAtomicUnit=on
  Out : Outport  VectorParamsAs1DForOutWhenUnconnected=off
  wires:
  Product1/1 -> Integrator/1  "Body Acceleration"
  Hydrostatics Forces/1(F_g) -> Sum2/1
  Coriolis & Centripetal Forces/1(F_C) -> Sum1/2
  Sum/1 -> Product1/2
  Sum2/1 -> Sum1/1
  Integrator/1 -> kinematics/1(nu), Damping Forces/1(Velocity), Coriolis & Centripetal Forces/1(Velocity)  "Body Velocity"
  In/1 -> Sum/1
  Sum1/1 -> Sum/2
  Damping Forces/1(F_Drag) -> Sum2/2
  Inverse of total mass/1 -> Product1/1
  kinematics/1(eta_dot) -> Mux/1, Integrator1/1  "Velocity"
  Integrator1/1 -> kinematics/2(eta), Mux/2, Hydrostatics Forces/1(Pose)  "Pose"
  Mux/1 -> Out/1

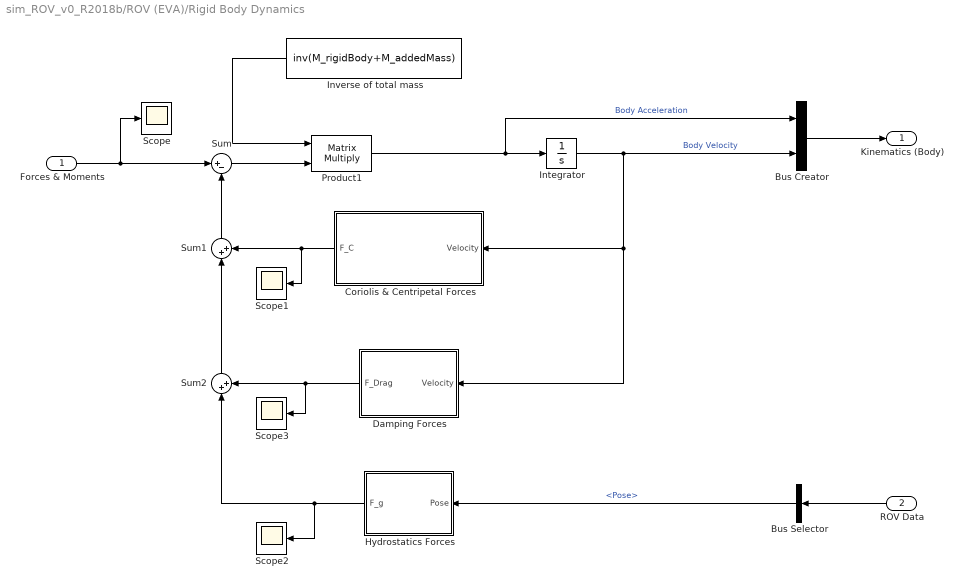
== system sim_ROV_v0_R2018b/ROV (EVA)/Rigid Body Dynamics ==
  Forces & Moments : Inport
  ROV Data : Inport  Port=2
  Bus Creator : BusCreator  Inputs=2
  Bus Selector : BusSelector  OutputSignals=Kinematics (Fixed).Pose
  Coriolis & Centripetal Forces : Subsystem
  Damping Forces : Subsystem
  Hydrostatics Forces : Subsystem
  Integrator : Integrator
  Inverse of total mass : Constant  Value=inv(M_rigidBody+M_addedMass)
  Product1 : Product  Multiplication=Matrix(*)  RndMeth=Zero
  Scope{,1..3} (4 alike) : Scope
  Sum : Sum  Inputs=|+-
  Sum1 : Sum  Inputs=|++
  Sum2 : Sum  Inputs=|++
  Kinematics (Body) : Outport  VectorParamsAs1DForOutWhenUnconnected=off
  wires:
  Inverse of total mass/1 -> Product1/1
  Sum1/1 -> Sum/2
  Sum2/1 -> Sum1/1
  Sum/1 -> Product1/2
  Damping Forces/1(F_Drag) -> Scope3/1, Sum2/2
  Hydrostatics Forces/1(F_g) -> Scope2/1, Sum2/1
  Coriolis & Centripetal Forces/1(F_C) -> Scope1/1, Sum1/2
  Forces & Moments/1 -> Scope/1, Sum/1
  Integrator/1 -> Damping Forces/1(Velocity), Coriolis & Centripetal Forces/1(Velocity), Bus Creator/2  "Body Velocity"
  Product1/1 -> Bus Creator/1, Integrator/1  "Body Acceleration"
  Bus Creator/1 -> Kinematics (Body)/1
  Bus Selector/1 -> Hydrostatics Forces/1(Pose)  "<Pose>"
  ROV Data/1 -> Bus Selector/1

== system sim_ROV_v0_R2018b/ROV (EVA)/Rigid Body Kinematics ==
  Kinematics (Body) : Inport
  Bus Creator : BusCreator  Inputs=3
  Bus Selector : BusSelector  OutputSignals=Body Velocity
  Derivative : Derivative
  Integrator : Integrator
  kinematics : MATLAB Function  TreatAsAtomicUnit=on
  Kinematics (Fixed) : Outport  VectorParamsAs1DForOutWhenUnconnected=off
  wires:
  Bus Selector/1 -> kinematics/1(nu)  "<Body Velocity>"
  Kinematics (Body)/1 -> Bus Selector/1
  Bus Creator/1 -> Kinematics (Fixed)/1
  Integrator/1 -> kinematics/2(eta), Bus Creator/3  "Pose"
  kinematics/1(eta_dot) -> Derivative/1, Bus Creator/2, Integrator/1  "Velocity"
  Derivative/1 -> Bus Creator/1  "Acceleration"

== system sim_ROV_v0_R2018b/Reference Generator/Step ==
  Step : Step  After=100  SampleTime=0
  Step1 : Step  Time=30  After=10  SampleTime=0
  Sum3 : Sum  Inputs=|+-
  step : Outport
  wires:
  Sum3/1 -> step/1
  Step1/1 -> Sum3/2
  Step/1 -> Sum3/1

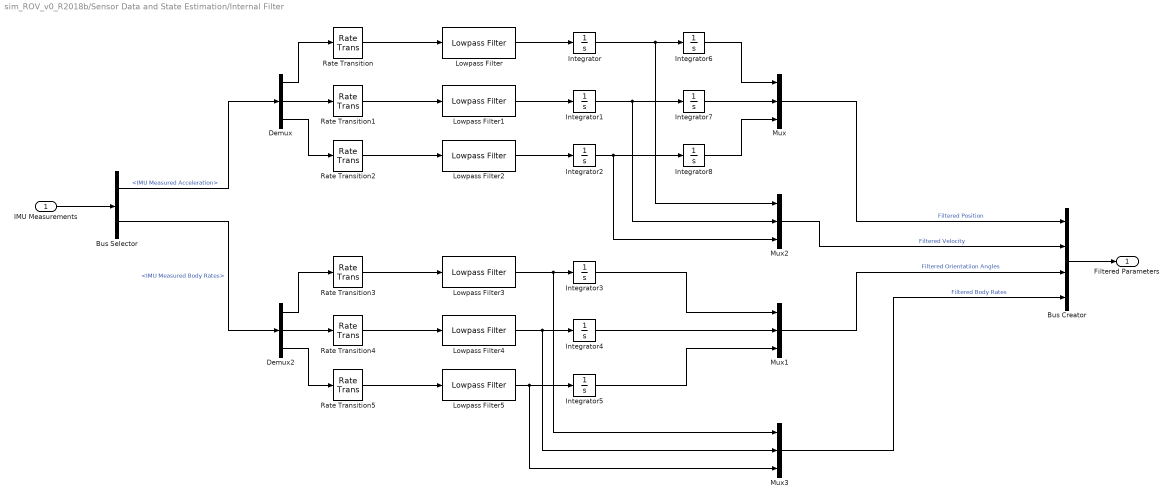
== system sim_ROV_v0_R2018b/Sensor Data and State Estimation/Internal Filter ==
  IMU Measurements : Inport
  Bus Creator : BusCreator  Inputs=4
  Bus Selector : BusSelector  OutputSignals=IMU Measured Acceleration,IMU Measured Body Rates
  Demux : Demux  Outputs=3
  Demux2 : Demux  Outputs=3
  Integrator{,1..8} (9 alike) : Integrator
  Lowpass Filter{,1..5} (6 alike) : dspfdesign/Lowpass Filter  FilterType=FIR  DesignForMinimumOrder=on  FilterOrder=50  PassbandFrequency=1/100  StopbandFrequency=45  PassbandRipple=0.1  StopbandAttenuation=80  SampleRateMode=Specify on dialog  SampleRate=100  SimulateUsing=Interpreted execution  roundingMode=Floor  coeffsDataTypeStr=fixdt(1,16)
  Mux{,1..3} (4 alike) : Mux  Inputs=3
  Rate Transition{,1..5} (6 alike) : RateTransition  OutPortSampleTime=Ts
  Filtered Parameters : Outport  VectorParamsAs1DForOutWhenUnconnected=off
  wires:
  Bus Selector/1 -> Demux/1  "<IMU Measured Acceleration>"
  IMU Measurements/1 -> Bus Selector/1
  Bus Selector/2 -> Demux2/1  "<IMU Measured Body Rates>"
  Demux/1 -> Rate Transition/1
  Demux/2 -> Rate Transition1/1
  Demux/3 -> Rate Transition2/1
  Demux2/2 -> Rate Transition4/1
  Demux2/3 -> Rate Transition5/1
  Demux2/1 -> Rate Transition3/1
  Rate Transition/1 -> Lowpass Filter/1
  Rate Transition1/1 -> Lowpass Filter1/1
  Rate Transition2/1 -> Lowpass Filter2/1
  Rate Transition3/1 -> Lowpass Filter3/1
  Rate Transition4/1 -> Lowpass Filter4/1
  Rate Transition5/1 -> Lowpass Filter5/1
  Lowpass Filter/1 -> Integrator/1
  Lowpass Filter1/1 -> Integrator1/1
  Lowpass Filter2/1 -> Integrator2/1
  Lowpass Filter3/1 -> Mux3/1, Integrator3/1
  Lowpass Filter4/1 -> Mux3/2, Integrator4/1
  Lowpass Filter5/1 -> Mux3/3, Integrator5/1
  Integrator/1 -> Mux2/1, Integrator6/1
  Integrator1/1 -> Mux2/2, Integrator7/1
  Integrator2/1 -> Mux2/3, Integrator8/1
  Integrator7/1 -> Mux/2
  Integrator8/1 -> Mux/3
  Integrator6/1 -> Mux/1
  Integrator4/1 -> Mux1/2
  Integrator3/1 -> Mux1/1
  Integrator5/1 -> Mux1/3
  Mux/1 -> Bus Creator/1  "Filtered Position"
  Mux2/1 -> Bus Creator/2  "Filtered Velocity"
  Mux1/1 -> Bus Creator/3  "Filtered Orientatiion Angles"
  Mux3/1 -> Bus Creator/4  "Filtered Body Rates"
  Bus Creator/1 -> Filtered Parameters/1

== system sim_ROV_v0_R2018b/Sensor Data and State Estimation/Sensor (IMU) ==
  IMU Inputs : Inport
  Bus Creator : BusCreator  Inputs=2
  Bus Selector : BusSelector  OutputSignals=IMU Data
  Demux : Demux  Outputs=5
  Three-axis Inertial Measurement Unit : aerolibnav/Three-axis Inertial Measurement Unit  units=Metric (MKS)  imu=[0 0 0]  i_Ts=0  dtype_a=on  w_a=190  z_a=0.707  a_sf_cc=[1 0 0; 0 1 0; 0 0 1]  a_bias=[0 0 0]  a_sat="[-inf  -inf  -inf  inf inf inf]"  dtype_g=on  w_g=190  z_g=0.707  g_sf_cc=[1 0 0; 0 1 0; 0 0 1]  g_bias=[0 0 0]  g_sens=[0 0 0]  g_sat="[-inf  -inf  -inf  inf inf inf]"  i_rand=on  i_seeds=[23093 23094 23095 23096 23097 23098]  i_pow=[0.00001 0.00001 0.00001 0.00001 0.00001 0.00001]
  IMU Measurements : Outport  VectorParamsAs1DForOutWhenUnconnected=off
  wires:
  Demux/1 -> Three-axis Inertial Measurement Unit/1
  Demux/5 -> Three-axis Inertial Measurement Unit/5
  Demux/4 -> Three-axis Inertial Measurement Unit/4
  Demux/2 -> Three-axis Inertial Measurement Unit/2
  Demux/3 -> Three-axis Inertial Measurement Unit/3
  Three-axis Inertial Measurement Unit/1 -> Bus Creator/1  "IMU Measured Acceleration"
  Three-axis Inertial Measurement Unit/2 -> Bus Creator/2  "IMU Measured Body Rates"
  Bus Selector/1 -> Demux/1  "<IMU Data>"
  IMU Inputs/1 -> Bus Selector/1
  Bus Creator/1 -> IMU Measurements/1

== system sim_ROV_v0_R2018b/Visualization/3D Animation ==
  Position : Inport
  "Roll, Pitch, Yaw" : Inport  Port=2
  3D Rotation : Subsystem
  Constant : Constant  Value=|
      | 2*[ 0        0         0
      |         2        0         0
      |         2        1.2       0
      |         0        1.2       0
      |         0        0         0
      |         0        0         1
      |         2        0         1
      |         2        1.2       1
      |         0        1.2       1
      |         0        0         1
      |         0        1.2       1
      |         0        1.2       0
      |         2        1.2       0
      |         2        1.2       1
      |         2        0         1
      |         2        0         0];
  MATLAB Function : MATLAB Function  TreatAsAtomicUnit=on
  wires:
  Constant/1 -> 3D Rotation/2(Points)
  "Roll, Pitch, Yaw"/1 -> 3D Rotation/1("Roll, Pitch, Yaw")
  Position/1 -> MATLAB Function/1(Position)
  3D Rotation/1(Transformed) -> MATLAB Function/2(srf_in)

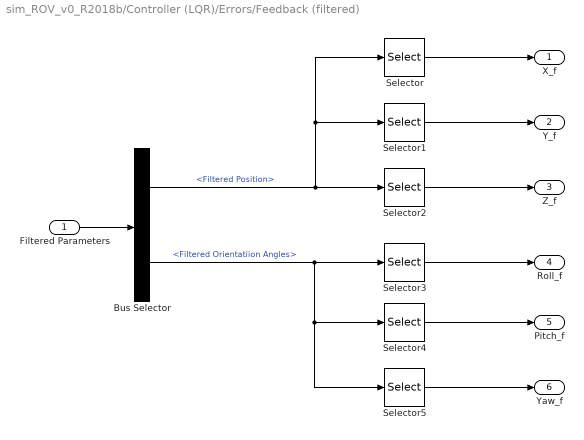
== system sim_ROV_v0_R2018b/Controller (LQR)/Errors/Feedback (filtered) ==
  Filtered Parameters : Inport
  Bus Selector : BusSelector  OutputSignals=Filtered Position,Filtered Orientatiion Angles
  Selector : Selector  InputPortWidth=3  IndexOptions=Index vector (dialog)  Indices=1  OutputSizes=1
  Selector1 : Selector  InputPortWidth=3  IndexOptions=Index vector (dialog)  Indices=2  OutputSizes=1
  Selector2 : Selector  InputPortWidth=3  IndexOptions=Index vector (dialog)  Indices=3  OutputSizes=1
  Selector3 : Selector  InputPortWidth=3  IndexOptions=Index vector (dialog)  Indices=1  OutputSizes=1
  Selector4 : Selector  InputPortWidth=3  IndexOptions=Index vector (dialog)  Indices=2  OutputSizes=1
  Selector5 : Selector  InputPortWidth=3  IndexOptions=Index vector (dialog)  Indices=3  OutputSizes=1
  X_f : Outport  VectorParamsAs1DForOutWhenUnconnected=off
  Y_f : Outport  Port=2  VectorParamsAs1DForOutWhenUnconnected=off
  Z_f : Outport  Port=3  VectorParamsAs1DForOutWhenUnconnected=off
  Roll_f : Outport  Port=4  VectorParamsAs1DForOutWhenUnconnected=off
  Pitch_f : Outport  Port=5  VectorParamsAs1DForOutWhenUnconnected=off
  Yaw_f : Outport  Port=6  VectorParamsAs1DForOutWhenUnconnected=off
  wires:
  Filtered Parameters/1 -> Bus Selector/1
  Bus Selector/1 -> Selector/1, Selector1/1, Selector2/1  "<Filtered Position>"
  Bus Selector/2 -> Selector3/1, Selector4/1, Selector5/1  "<Filtered Orientatiion Angles>"
  Selector/1 -> X_f/1
  Selector1/1 -> Y_f/1
  Selector2/1 -> Z_f/1
  Selector3/1 -> Roll_f/1
  Selector4/1 -> Pitch_f/1
  Selector5/1 -> Yaw_f/1

== system sim_ROV_v0_R2018b/Controller (LQR)/Errors/Reference Signals ==
  Reference : Inport
  Demux : Demux  Outputs=6
  X_ref : Outport  VectorParamsAs1DForOutWhenUnconnected=off
  Y_ref : Outport  Port=2  VectorParamsAs1DForOutWhenUnconnected=off
  Z_ref : Outport  Port=3  VectorParamsAs1DForOutWhenUnconnected=off
  Roll_ref : Outport  Port=4  VectorParamsAs1DForOutWhenUnconnected=off
  Pitch_ref : Outport  Port=5  VectorParamsAs1DForOutWhenUnconnected=off
  Yaw_ref : Outport  Port=6  VectorParamsAs1DForOutWhenUnconnected=off
  wires:
  Reference/1 -> Demux/1
  Demux/5 -> Pitch_ref/1
  Demux/4 -> Roll_ref/1
  Demux/3 -> Z_ref/1
  Demux/2 -> Y_ref/1
  Demux/6 -> Yaw_ref/1
  Demux/1 -> X_ref/1

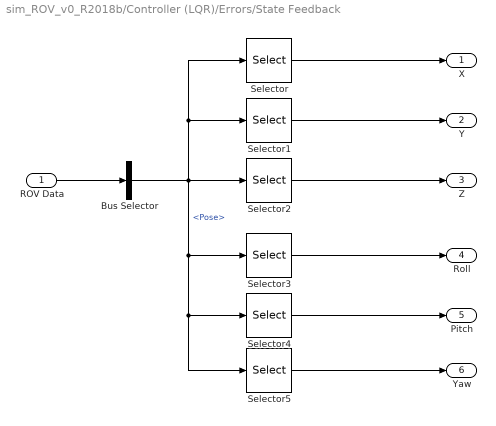
== system sim_ROV_v0_R2018b/Controller (LQR)/Errors/State Feedback ==
  ROV Data : Inport
  Bus Selector : BusSelector  OutputSignals=Kinematics (Fixed).Pose
  Selector : Selector  InputPortWidth=6  IndexOptions=Index vector (dialog)  Indices=1  OutputSizes=1
  Selector1 : Selector  InputPortWidth=6  IndexOptions=Index vector (dialog)  Indices=2  OutputSizes=1
  Selector2 : Selector  InputPortWidth=6  IndexOptions=Index vector (dialog)  Indices=3  OutputSizes=1
  Selector3 : Selector  InputPortWidth=6  IndexOptions=Index vector (dialog)  Indices=4  OutputSizes=1
  Selector4 : Selector  InputPortWidth=6  IndexOptions=Index vector (dialog)  Indices=5  OutputSizes=1
  Selector5 : Selector  InputPortWidth=6  IndexOptions=Index vector (dialog)  Indices=6  OutputSizes=1
  X : Outport  VectorParamsAs1DForOutWhenUnconnected=off
  Y : Outport  Port=2  VectorParamsAs1DForOutWhenUnconnected=off
  Z : Outport  Port=3  VectorParamsAs1DForOutWhenUnconnected=off
  Roll : Outport  Port=4  VectorParamsAs1DForOutWhenUnconnected=off
  Pitch : Outport  Port=5  VectorParamsAs1DForOutWhenUnconnected=off
  Yaw : Outport  Port=6  VectorParamsAs1DForOutWhenUnconnected=off
  wires:
  ROV Data/1 -> Bus Selector/1
  Bus Selector/1 -> Selector5/1, Selector4/1, Selector3/1, Selector2/1, Selector1/1, Selector/1  "<Pose>"
  Selector4/1 -> Pitch/1
  Selector3/1 -> Roll/1
  Selector2/1 -> Z/1
  Selector1/1 -> Y/1
  Selector5/1 -> Yaw/1
  Selector/1 -> X/1

== system sim_ROV_v0_R2018b/Controller (LQR)/Test/Chirp ==
  Chirp Signal : simulink/Sources/Chirp Signal  f1=0.005  T=sim_time  f2=1
  Gain : Gain  Gain=80
  chirp : Outport  VectorParamsAs1DForOutWhenUnconnected=off
  wires:
  Chirp Signal/1 -> Gain/1
  Gain/1 -> chirp/1

== system sim_ROV_v0_R2018b/Controller (LQR)/Test/Impulse ==
  Derivative : Derivative
  Gain : Gain  Gain=0.001
  Step2 : Step  SampleTime=0
  impulse : Outport
  wires:
  Step2/1 -> Derivative/1
  Derivative/1 -> Gain/1
  Gain/1 -> impulse/1
